simulink model "Single_Lag_Adjoint_simu"  (R2024b)
settings: Solver=VariableStepAuto  StartTime=0.0  StopTime=10.0  RelTol=1e-3
PreLoadFcn:
  | load("Single Lag Adjoint Results.mat")
values from neighbouring files (symbols this model uses):
  p =     [Single Lag Adjoint Results.mat]
settings Model: Creator=benme  LastModifiedBy=benme

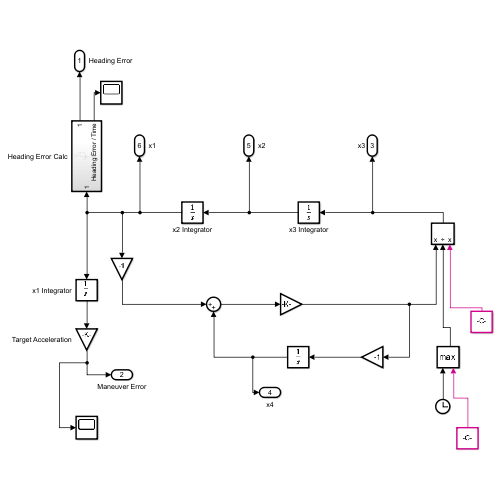
[thumbnail: Simulink's stored preview of the top-level diagram]
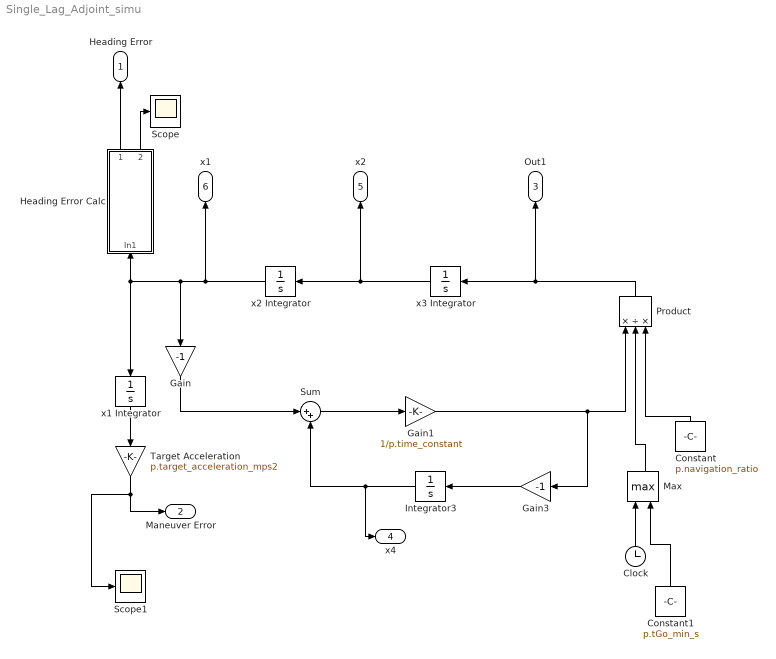
== system Single_Lag_Adjoint_simu ==
  Clock : Clock
  Constant : Constant  Value=p.navigation_ratio
  Constant1 : Constant  Value=p.tGo_min_s
  Gain : Gain  Gain=-1
  Gain1 : Gain  Gain=1/p.time_constant
  Gain3 : Gain  Gain=-1
  Heading Error Calc : Subsystem
  Integrator3 : Integrator
  Max : MinMax  Function=max  Inputs=2
  Product : Product  Inputs=*/*
  Scope : Scope
  Scope1 : Scope
  Sum : Sum  Inputs=|++
  Target Acceleration : Gain  Gain=p.target_acceleration_mps2
  x1 Integrator : Integrator
  x2 Integrator : Integrator
  x3 Integrator : Integrator  InitialCondition=1
  Heading Error : Outport
  Maneuver Error : Outport  Port=2
  Out1 : Outport  Port=3  SignalName=x3
  x4 : Outport  Port=4
  x2 : Outport  Port=5
  x1 : Outport  Port=6
  wires:
  x3 Integrator/1 -> x2 Integrator/1, x2/1
  x2 Integrator/1 -> Gain/1, Heading Error Calc/1(In1), x1 Integrator/1, x1/1
  Heading Error Calc/1(Out1) -> Heading Error/1
  x1 Integrator/1 -> Target Acceleration/1
  Target Acceleration/1 -> Scope1/1, Maneuver Error/1
  Gain/1 -> Sum/1
  Integrator3/1 -> x4/1, Sum/2
  Sum/1 -> Gain1/1
  Gain1/1 -> Product/1, Gain3/1
  Gain3/1 -> Integrator3/1
  Clock/1 -> Max/1
  Constant/1 -> Product/3
  Heading Error Calc/2(Heading Error / Time) -> Scope/1
  Product/1 -> x3 Integrator/1, Out1/1
  Constant1/1 -> Max/2
  Max/1 -> Product/2

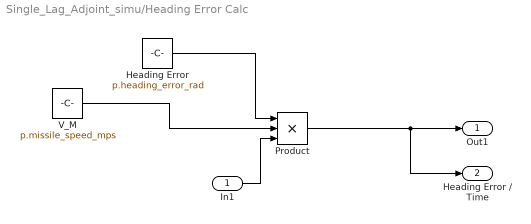
== system Single_Lag_Adjoint_simu/Heading Error Calc ==
  In1 : Inport
  Heading Error : Constant  Value=p.heading_error_rad
  Product : Product  Inputs=3
  V_M : Constant  Value=p.missile_speed_mps
  Out1 : Outport
  Heading Error / Time : Outport  Port=2
  wires:
  In1/1 -> Product/3
  Heading Error/1 -> Product/1
  V_M/1 -> Product/2
  Product/1 -> Heading Error / Time/1, Out1/1
